simulink model "CTRL_LO_ST1_test"  (R2023b)
settings: Solver=VariableStepAuto  StartTime=0.0  StopTime=10.0  RelTol=1e-3
libraries: CTRL_LO_ST1 x1
settings Model: Creator=blatak  LastModifiedBy=blatak

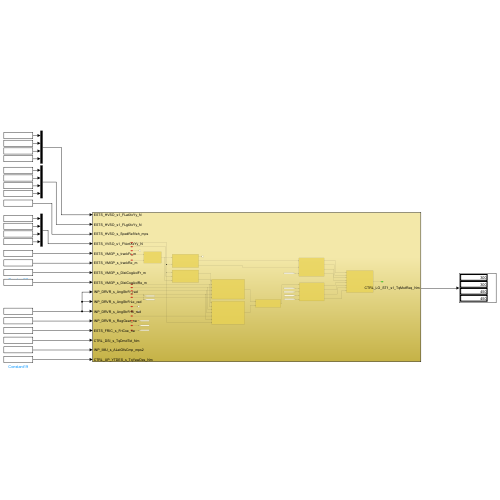
[thumbnail: Simulink's stored preview of the top-level diagram]
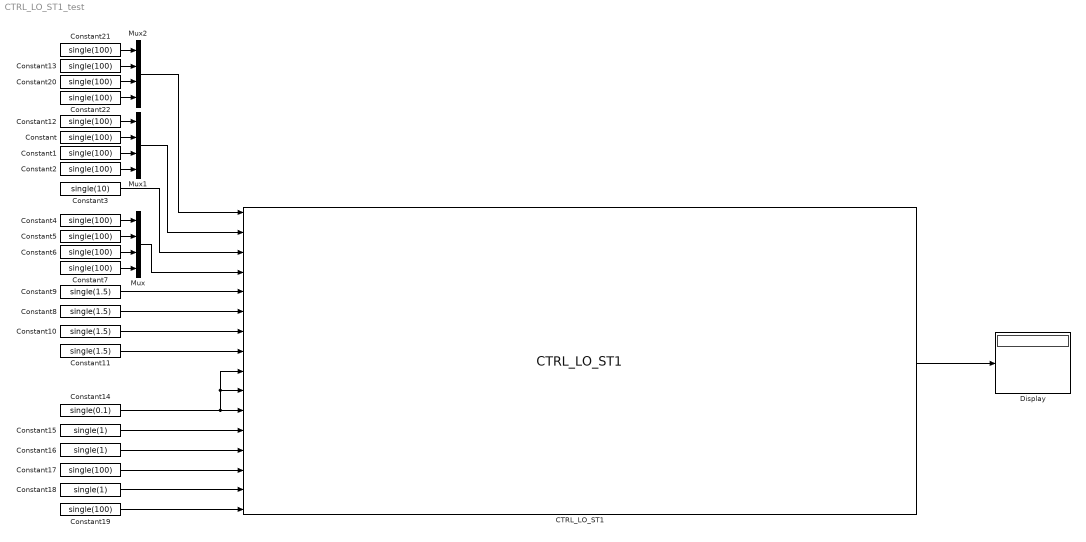
== system CTRL_LO_ST1_test ==
  CTRL_LO_ST1 : CTRL_LO_ST1/CTRL_LO_ST1  SystemSampleTime=-1  VariantActivationTime=update diagram  AllowFlexibleInterface=on  Latency=0  AutoFrameSizeCalculation=off
  Constant{,1..2,4..7,12..13,17,19..22} (14 alike) : Constant  Value=single(100)
  Constant{8..11} (4 alike) : Constant  Value=single(1.5)
  Constant14 : Constant  Value=single(0.1)
  Constant15 : Constant  Value=single(1)
  Constant16 : Constant  Value=single(1)
  Constant18 : Constant  Value=single(1)
  Constant3 : Constant  Value=single(10)
  Display : Display
  Mux : Mux
  Mux1 : Mux
  Mux2 : Mux
  wires:
  Constant19/1 -> CTRL_LO_ST1/16
  Constant18/1 -> CTRL_LO_ST1/15
  Constant17/1 -> CTRL_LO_ST1/14
  Constant16/1 -> CTRL_LO_ST1/13
  Constant15/1 -> CTRL_LO_ST1/12
  Constant14/1 -> CTRL_LO_ST1/9, CTRL_LO_ST1/10, CTRL_LO_ST1/11
  Constant11/1 -> CTRL_LO_ST1/8
  Constant10/1 -> CTRL_LO_ST1/7
  Constant8/1 -> CTRL_LO_ST1/6
  Constant9/1 -> CTRL_LO_ST1/5
  Constant4/1 -> Mux/1
  Constant5/1 -> Mux/2
  Constant6/1 -> Mux/3
  Constant7/1 -> Mux/4
  Mux/1 -> CTRL_LO_ST1/4
  Constant3/1 -> CTRL_LO_ST1/3
  Constant12/1 -> Mux1/1
  Constant/1 -> Mux1/2
  Constant1/1 -> Mux1/3
  Constant2/1 -> Mux1/4
  Constant20/1 -> Mux2/3
  Constant21/1 -> Mux2/1
  Constant22/1 -> Mux2/4
  Constant13/1 -> Mux2/2
  Mux1/1 -> CTRL_LO_ST1/2
  Mux2/1 -> CTRL_LO_ST1/1
  CTRL_LO_ST1/1 -> Display/1
